simulink model "lab5"  (R2021a)
settings: Solver=VariableStepAuto  StartTime=0.0  StopTime=10.0  RelTol=1e-3
settings Model: Creator=vedve  LastModifiedBy=vedve

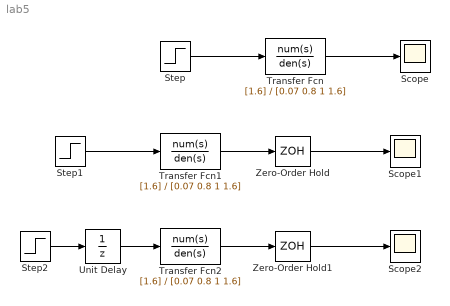
== system lab5 ==
  Scope : Scope
  Scope1 : Scope
  Scope2 : Scope
  Step : Step  SampleTime=0
  Step1 : Step  SampleTime=0
  Step2 : Step  SampleTime=0
  Transfer Fcn : TransferFcn  Numerator=[1.6]  Denominator=[0.07 0.8 1 1.6]
  Transfer Fcn1 : TransferFcn  Numerator=[1.6]  Denominator=[0.07 0.8 1 1.6]
  Transfer Fcn2 : TransferFcn  Numerator=[1.6]  Denominator=[0.07 0.8 1 1.6]
  Unit Delay : UnitDelay  SampleTime=2  HasFrameUpgradeWarning=on
  Zero-Order Hold : ZeroOrderHold  SampleTime=0.5
  Zero-Order Hold1 : ZeroOrderHold  SampleTime=0.5
  wires:
  Step/1 -> Transfer Fcn/1
  Transfer Fcn/1 -> Scope/1
  Step1/1 -> Transfer Fcn1/1
  Transfer Fcn1/1 -> Zero-Order Hold/1
  Zero-Order Hold/1 -> Scope1/1
  Zero-Order Hold1/1 -> Scope2/1
  Transfer Fcn2/1 -> Zero-Order Hold1/1
  Step2/1 -> Unit Delay/1
  Unit Delay/1 -> Transfer Fcn2/1
